simulink model "zadanie3"  (Simulink 6.3)
settings: Solver=ode3  StartTime=0.0  StopTime=20.0  FixedStep=0.01  RelTol=1e-3
settings Model: LastModifiedBy=Umka

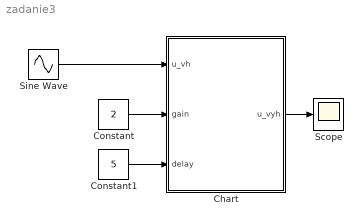
== system zadanie3 ==
  Chart : Stateflow chart
  Constant : Constant  Value=2
  Constant1 : Constant  Value=5
  Scope : Scope
      settings: YMin=-2  YMax=2
  Sine Wave : Sin  SampleTime=0
  wires:
  Sine Wave/1 -> Chart/1(u_vh)
  Constant/1 -> Chart/2(gain)
  Constant1/1 -> Chart/3(delay)
  Chart/1(u_vyh) -> Scope/1

== stateflow chart Chart ==
  state A
    u_vyh = 0;
  state B
    du: u_vyh = gain*u_vh;
  A -> B : [t>delay]
  (default) -> A
  data: u_vh input double; gain input double; delay input double; u_vyh output double
